simulink model "map_usage"  (R2024b)
settings: Solver=ode1  StartTime=0.0  StopTime=inf  FixedStep=0.01  RelTol=1e-3  EnableMultiTasking=on
PostLoadFcn:
  | qlabs_setup
model workspace (MAT data in the model file):
  Sig = Simulink.Signal
  Sig.Dimensions = -1
  Sig.DimensionsMode = 'auto'
  Sig.Complexity = 'auto'
  Sig.SampleTime = -1
  Sig.SamplingMode = 'auto'
  Sig.DataType = 'auto'
  downCamStepSize = Simulink.Parameter
  downCamStepSize.Value = Simulink.data.Expression
  downCamStepSize.Value.ExpressionString = "qc_get_step_size*ceil(1/30/qc_get_step_size)"
  downCamStepSize.Complexity = 'real'
  downCamStepSize.Dimensions = -1
  downCamStepSize.DataType = 'auto'
  lidarStepSize = Simulink.Parameter
  lidarStepSize.Value = Simulink.data.Expression
  lidarStepSize.Value.ExpressionString = "qc_get_step_size*ceil(1/5/qc_get_step_size)"
  lidarStepSize.Complexity = 'real'
  lidarStepSize.Dimensions = -1
  lidarStepSize.DataType = 'auto'
  mainStepSize = Simulink.Parameter
  mainStepSize.Value = Simulink.data.Expression
  mainStepSize.Value.ExpressionString = "qc_get_step_size"
  mainStepSize.Complexity = 'real'
  mainStepSize.Dimensions = -1
  mainStepSize.DataType = 'auto'
  mode = Simulink.Parameter
  mode.Value = 2
  mode.Complexity = 'real'
  mode.Dimensions = [1 1]
  mode.Description = '0 - education speeds via wheel speed commands
    | 1 - education speeds via body speed commands
    | 2 - research speeds via wheel speed commands
    | 3 - research speeds via body speed commands'
  mode.DataType = 'auto'
  realSenseStepSize = Simulink.Parameter
  realSenseStepSize.Value = Simulink.data.Expression
  realSenseStepSize.Value.ExpressionString = "qc_get_step_size*ceil(1/30/qc_get_step_size)"
  realSenseStepSize.Complexity = 'real'
  realSenseStepSize.Dimensions = -1
  realSenseStepSize.DataType = 'auto'
values from neighbouring files (symbols this model uses):
  map = zeros(mapHeight*pointPerMeter, mapWidth*pointPerMeter)    [map_creator.m]    (also in map_creator_real.m)
  obstacles = [obstacles; coordinateX, coordinateY, rayon;]    [init.m]    (also in init1.m; init_V2.m; init_V3.m; map_creator.m = [)
  pointPerMeter = 50    [map_creator.m]    (also in map_creator_real.m)
  waypoints = [ ... (first row only)    [init.m]    (also in init1.m; init_V2.m; init_V3.m)
undefined symbols (not defined in the file or in its folder): Point
libraries: quarc_library x9, simulink_extras x2
settings Model: ExtModeTrigDuration=10000  Creator=mbohra  LastModifiedBy=simon
settings SolverCC: PositivePriorityOrder=on  AutoInsertRateTranBlk=on
settings DebuggingCC: UnderspecifiedInitializationDetection=Classic  MergeDetectMultiDrivingBlocksExec=none
settings ModelReferenceCC: PropagateSignalLabelsOutOfModel=off
settings RTWCC: Description=QUARC Win64 Target Using Toolchain  SystemTargetFile=quarc_win64.tlc  Toolchain=QUARC win64 | nmake (64-bit Windows)  BuildConfiguration=Faster Runs  GPUComputeCapability=3.5
settings STFCustomTargetCC: TargetLangStandard=C99 (ISO)  ConcurrentExecutionCompliant=on  GRTInterface=on  UseToolchainInfoCompliant=on  SystemTargetFile=quarc_win64.tlc
settings GRTTargetCC: ParMdlRefBuildCompliant=off  CompOptLevelCompliant=off  CombineOutputUpdateFcns=off  MatFileLogging=off  CPPClassGenCompliant=off  GRTInterface=on  ExtMode=on  ExtModeMexFile=quarc_comm

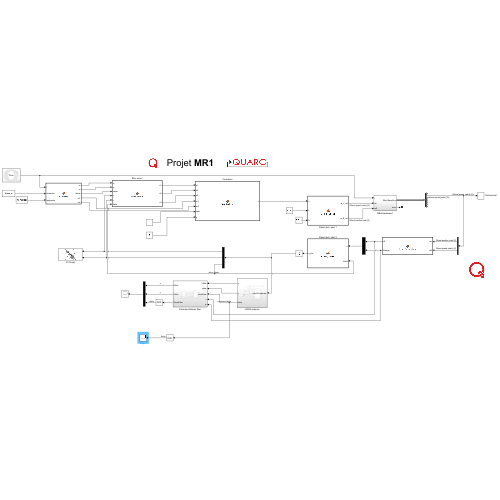
[thumbnail: Simulink's stored preview of the top-level diagram]
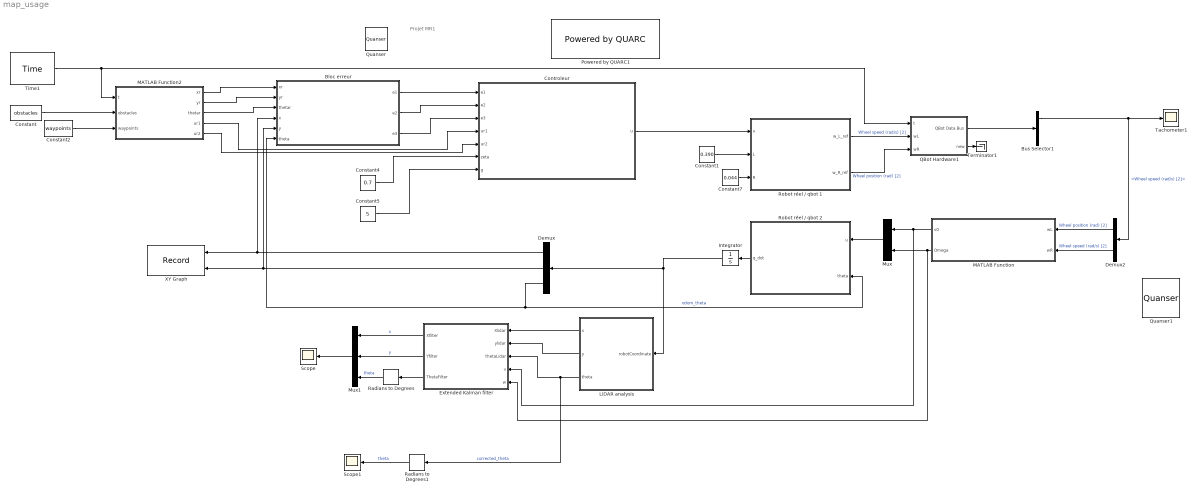
== system map_usage ==
  note: Projet MR1
  Bloc erreur : MATLAB Function  TreatAsAtomicUnit=on
  Bus Selector1 : BusSelector  OutputSignals=Wheel position (rad) [2],Wheel speed (rad/s) [2],Motor Cmd (Volts) [2],Acceleration (m/s/s) [3],Gyroscope (rad/s) [3],Current (Amps) [2],Battery (Volts)
  Constant : Constant  Value=obstacles
  Constant1 : Constant  Value=0.390
  Constant2 : Constant  Value=waypoints
  Constant4 : Constant  Value=0.7
  Constant5 : Constant  Value=5
  Constant7 : Constant  Value=0.044
  Controleur : MATLAB Function  TreatAsAtomicUnit=on
  Demux : Demux  Outputs=3
  Demux2 : Demux  Outputs=2
  Extended Kalman filter : Subsystem
  Integrator : Integrator
  LiDAR analysis : Subsystem
  MATLAB Function : MATLAB Function  TreatAsAtomicUnit=on
  MATLAB Function2 : MATLAB Function  TreatAsAtomicUnit=on
  Mux : Mux  Inputs=2
  Mux1 : Mux  Inputs=3
  Powered by QUARC1 : quarc_library/Logos/Powered by QUARC
  QBot Hardware1 : Subsystem
  Quanser : quarc_library/Logos/Quanser
  Quanser1 : quarc_library/Logos/Quanser
  Radians to Degrees : simulink_extras/Transformations/Radians to Degrees
  Radians to Degrees1 : simulink_extras/Transformations/Radians to Degrees
  Robot réel / qbot 1 : MATLAB Function  TreatAsAtomicUnit=on
  Robot réel / qbot 2 : MATLAB Function  TreatAsAtomicUnit=on
  Scope : Scope
  Scope1 : Scope
  Tachometer1 : Scope
  Terminator1 : Terminator
  Time1 : quarc_library/Sources/Time/Time  time_source=Wall clock  sample_time=qc_get_step_size
  XY Graph : Record  FileSettingsInternal="{\"entries\":[{\"content\":{\"excelSettings\":{\"content\":{},\"type\":\"Streamout.ExcelSettings\"}},\"type\":\"Streamout.FileSettingStorage\",\"uuid\":\"\"}],\"packageUris\":[\"http:\\/\\/schema.mathworks.com\\/mf0\\/streamout_blocks\\/R2020a\"],\"version\":\"1.0\"}"  Layout=[1 1]  SignalsInternal="{\"entries\":[{\"content\":{\"signals\":[{\"content\":{\"blockPath\":[],\"dimensions\":[1,1],\"domain\":\"\",\"lineColor\":\"#a2142f\",\"plots\":[ 1 ],\"port\":1,\"signalID\":1,\"signalName\":\"Demux:1\"},\"type\":\"RecordBlkView.Signal\",\"uuid\":\"\"},{\"content\":{\"blockPath\":[],\"dimensions\":[1,1],\"domain\":\"\",\"lineColor\":\"#139fff\",\"plots\":[ 1 ],\"port\":2,\"signalID\":2,\"signalName\":\"Demux:2\"},\"type\":\"RecordBlkView.Signal\",\"uuid\":\"\"}]},\"type\":\"RecordBlkView.InputSignals\",\"uuid\":\"\"}],\"packageUris\":[\"http:\\/\\/schema.mathworks.com\\/mf0\\/streamout_blocks\\/R2020a\"],\"version\":\"1.0\"}"  VisualizationBindings="{\"xyplotplugin\":{\"info\":[{\"series\":[{\"bindingParametersList\":[{\"parameter\":\"X-Axis\",\"signalID\":1,\"signalName\":\"Demux:1\"},{\"parameter\":\"Y-Axis\",\"signalID\":2,\"signalName\":\"Demux:2\"}],\"seriesID\":0}],\"subplotID\":1}]}}"  CompatibilityTag=XY
  wires:
  Controleur/1(u) -> Robot réel / qbot 1/1(u)
  Constant4/1 -> Controleur/6(zeta)
  Demux/3 -> Robot réel / qbot 2/2(theta), Bloc erreur/6(theta)  "odom_theta"
  Robot réel / qbot 2/1(q_dot) -> Integrator/1
  Bloc erreur/1(e1) -> Controleur/1(e1)
  Demux2/1 -> MATLAB Function/1(wL)  "Wheel position (rad) [2]"
  Demux2/2 -> MATLAB Function/2(wR)  "Wheel speed (rad/s) [2]"
  MATLAB Function/2(Omega) -> Extended Kalman filter/5(w), Mux/2
  Constant1/1 -> Robot réel / qbot 1/2(L)
  Robot réel / qbot 1/1(w_L_ref) -> QBot Hardware1/2(wL)  "Wheel speed (rad/s) [2]"
  Constant5/1 -> Controleur/7(g)
  MATLAB Function2/4(ur1) -> Controleur/4(ur1)
  Time1/1 -> QBot Hardware1/1(t), MATLAB Function2/1(t)
  MATLAB Function/1(v0) -> Extended Kalman filter/4(v), Mux/1
  QBot Hardware1/2(new) -> Terminator1/1
  Bus Selector1/2 -> Demux2/1, Tachometer1/1  "<Wheel speed (rad/s) [2]>"
  MATLAB Function2/1(xr) -> Bloc erreur/1(xr)
  MATLAB Function2/5(ur2) -> Controleur/5(ur2)
  Integrator/1 -> LiDAR analysis/1(robotCoordinate), Demux/1
  Bloc erreur/2(e2) -> Controleur/2(e2)
  Bloc erreur/3(e3) -> Controleur/3(e3)
  Demux/1 -> Bloc erreur/4(x), XY Graph/1
  QBot Hardware1/1(QBot Data Bus) -> Bus Selector1/1
  Robot réel / qbot 1/2(w_R_ref) -> QBot Hardware1/3(wR)  "Wheel position (rad) [2]"
  Constant7/1 -> Robot réel / qbot 1/3(R)
  MATLAB Function2/2(yr) -> Bloc erreur/2(yr)
  MATLAB Function2/3(thetar) -> Bloc erreur/3(thetar)
  Mux/1 -> Robot réel / qbot 2/1(u)
  Constant/1 -> MATLAB Function2/2(obstacles)
  Constant2/1 -> MATLAB Function2/3(waypoints)
  Demux/2 -> Bloc erreur/5(y), XY Graph/2
  LiDAR analysis/1(x) -> Extended Kalman filter/1(Xlidar)
  LiDAR analysis/2(y) -> Extended Kalman filter/2(ylidar)
  LiDAR analysis/3(theta) -> Radians to Degrees1/1, Extended Kalman filter/3(thetaLidar)  "corrected_theta"
  Extended Kalman filter/1(Xfilter) -> Mux1/1  "x"
  Extended Kalman filter/2(Yfilter) -> Mux1/2  "y"
  Extended Kalman filter/3(ThetaFilter) -> Radians to Degrees/1
  Mux1/1 -> Scope/1
  Radians to Degrees/1 -> Mux1/3  "theta"
  Radians to Degrees1/1 -> Scope1/1  "theta"

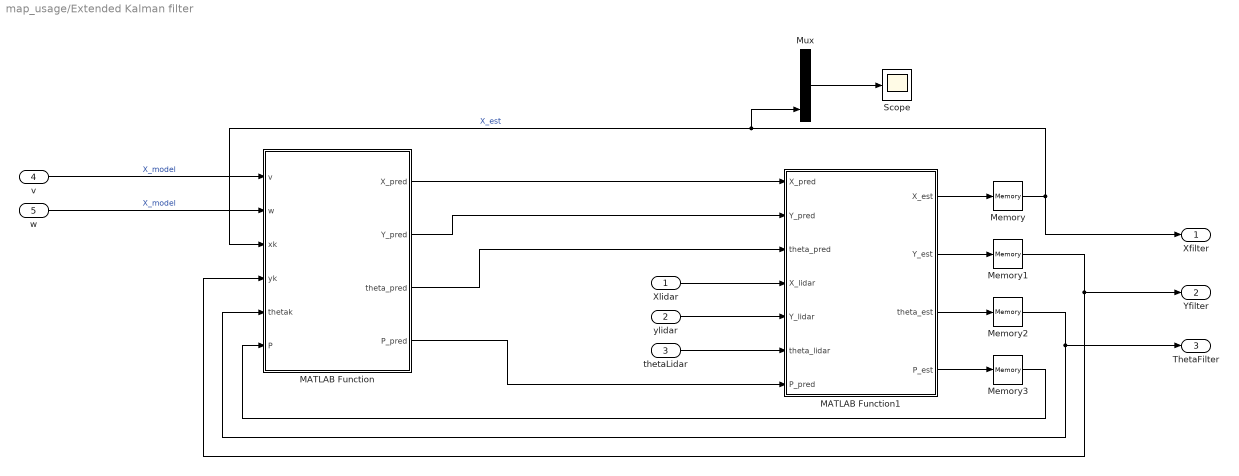
== system map_usage/Extended Kalman filter ==
  Xlidar : Inport
  ylidar : Inport  Port=2
  thetaLidar : Inport  Port=3
  v : Inport  Port=4
  w : Inport  Port=5
  MATLAB Function : MATLAB Function  TreatAsAtomicUnit=on
  MATLAB Function1 : MATLAB Function  TreatAsAtomicUnit=on
  Memory{,1..3} (4 alike) : Memory
  Mux : Mux  Inputs=3
  Scope : Scope
  Xfilter : Outport
  Yfilter : Outport  Port=2
  ThetaFilter : Outport  Port=3
  wires:
  MATLAB Function1/3(theta_est) -> Memory2/1
  MATLAB Function/2(Y_pred) -> MATLAB Function1/2(Y_pred)
  MATLAB Function1/4(P_est) -> Memory3/1
  MATLAB Function/1(X_pred) -> MATLAB Function1/1(X_pred)
  Memory/1 -> Mux/3, MATLAB Function/3(xk), Xfilter/1  "X_est"
  Memory2/1 -> MATLAB Function/5(thetak), ThetaFilter/1
  MATLAB Function1/1(X_est) -> Memory/1
  MATLAB Function/4(P_pred) -> MATLAB Function1/7(P_pred)
  MATLAB Function/3(theta_pred) -> MATLAB Function1/3(theta_pred)
  v/1 -> MATLAB Function/1(v)  "X_model"
  Memory3/1 -> MATLAB Function/6(P)
  Memory1/1 -> MATLAB Function/4(yk), Yfilter/1
  MATLAB Function1/2(Y_est) -> Memory1/1
  Mux/1 -> Scope/1
  Xlidar/1 -> MATLAB Function1/4(X_lidar)
  ylidar/1 -> MATLAB Function1/5(Y_lidar)
  thetaLidar/1 -> MATLAB Function1/6(theta_lidar)
  w/1 -> MATLAB Function/2(w)  "X_model"

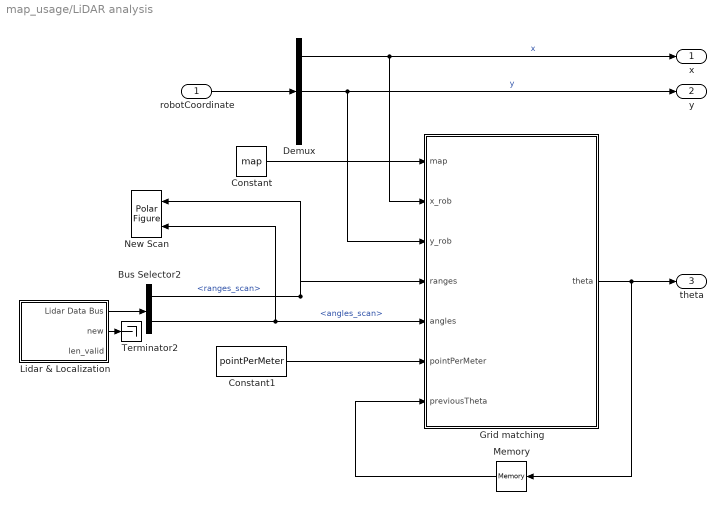
== system map_usage/LiDAR analysis ==
  robotCoordinate : Inport
  Bus Selector2 : BusSelector  OutputSignals=ranges_scan,angles_scan
  Constant : Constant  Value=map
  Constant1 : Constant  Value=pointPerMeter
  Demux : Demux  Outputs=3
  Grid matching : MATLAB Function  TreatAsAtomicUnit=on
  Lidar & Localization : Subsystem
  Memory : Memory
  New Scan : quarc_library/Sinks/Figures/Polar Figure  figure_mode=Use figure window  figure_tag=figure1  axes_tag=axes1  plot_mode=Frame-based  minimum_rho=0  maximum_rho=4  minimum_theta=0  maximum_theta=360  zero_location=top  direction=counterclockwise  buffer_size=1  update_rate=1  sample_time=-1  initial_position="520  231  433  389"  initial_visibility=off  line1_style=None  line1_width=0.5  line1_color=[0 0.4470 0.7410]  marker1=Point (.)  marker1_size=6  marker1_edge_color=[0 0.447059 0.741176]  marker1_face_color=[0 0.447059 0.741176]  line2_style=Solid line (-)  line2_width=0.5  line2_color=[0.85098 0.32549 0.0980392]  marker2=None  marker2_size=6  marker2_edge_color=[0.85098 0.32549 0.0980392]  marker2_face_color=[0.85098 0.32549 0.0980392]  line3_style=Solid line (-)  line3_width=0.5  line3_color=[0.929412 0.694118 0.12549]  marker3=None  marker3_size=6  marker3_edge_color=[0.929412 0.694118 0.12549]  marker3_face_color=[0.929412 0.694118 0.12549]  line4_style=Solid line (-)  line4_width=0.5  line4_color=[0.494118 0.184314 0.556863]  marker4=None  marker4_size=6  marker4_edge_color=[0.494118 0.184314 0.556863]  marker4_face_color=[0.494118 0.184314 0.556863]  line5_style=Solid line (-)  line5_width=0.5  line5_color=[0.466667 0.67451 0.188235]  marker5=None  marker5_size=6  marker5_edge_color=[0.466667 0.67451 0.188235]  marker5_face_color=[0.466667 0.67451 0.188235]
      settings: SourceProductName=QUARC Targets
  Terminator2 : Terminator
  x : Outport
  y : Outport  Port=2
  theta : Outport  Port=3
  wires:
  Constant/1 -> Grid matching/1(map)
  Demux/2 -> Grid matching/3(y_rob), y/1  "y"
  Demux/1 -> Grid matching/2(x_rob), x/1  "x"
  robotCoordinate/1 -> Demux/1
  Grid matching/1(theta) -> theta/1, Memory/1
  Lidar & Localization/1(Lidar Data Bus) -> Bus Selector2/1
  Lidar & Localization/2(new) -> Terminator2/1
  Bus Selector2/2 -> Grid matching/5(angles), New Scan/2  "<angles_scan>"
  Bus Selector2/1 -> Grid matching/4(ranges), New Scan/1  "<ranges_scan>"
  Constant1/1 -> Grid matching/6(pointPerMeter)
  Memory/1 -> Grid matching/7(previousTheta)

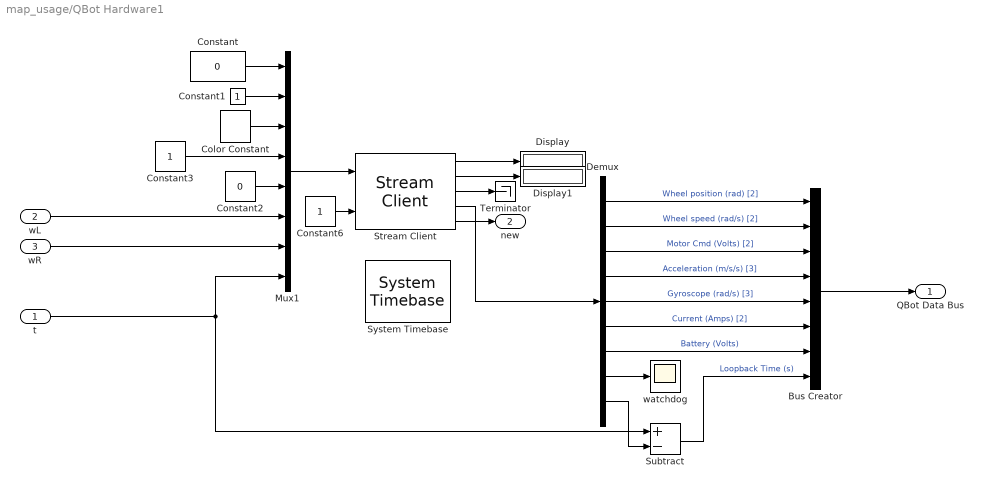
== system map_usage/QBot Hardware1 ==
  t : Inport
  wL : Inport  Port=2
  wR : Inport  Port=3
  Bus Creator : BusCreator  Inputs=8
  Color Constant : quarc_library/Sources/Signals/Color Constant  color=[1 0.07451 0.65098]
      settings: SourceProductName=QUARC Targets
  Constant : Constant  Value=0
  Constant1 : Constant
  Constant2 : Constant  Value=0
  Constant3 : Constant
  Constant6 : Constant
  Demux : Demux  Outputs=[2 2 2 3 3 2 1 1 1]
  Display : Display
  Display1 : Display
  Mux1 : Mux  Inputs=8
  Stream Client : quarc_library/Communications/Basic/Stream Client  uri_source=Specify via dialog (do not evaluate)  uri=tcpip://localhost:18888  send_buffer_size=1460  receive_buffer_size=1460  byte_order=little endian (Intel - LSB first)  optimization=Minimum latency  send_options=Send most recent data  receive_options=Receive most recent data  default_value=zeros(17,1)  sample_time=qc_get_step_size  active=on  implementation=Use blocking I/O in a separate thread  send_fifo_size=1000  receive_fifo_size=1000  send_priority=0  receive_priority=0  send_dimensions=off  receive_dimensions=off  max_dimensions=-1  data_type=Inherited via back propagation  type_expr=BusObject
      settings: AttributesFormatString="\"tcpip://localhost:18888\""
  Subtract : Sum  Inputs=+-
  System Timebase : quarc_library/Advanced/Timing/System Timebase  stop_on_overrun=off
      settings: SourceProductName=QUARC Targets
  Terminator : Terminator
  watchdog : Scope
  QBot Data Bus : Outport
  new : Outport  Port=2
  wires:
  Demux/2 -> Bus Creator/2  "Wheel speed (rad/s) [2]"
  Constant/1 -> Mux1/1
  Stream Client/3 -> Terminator/1
  Stream Client/1 -> Display/1
  Constant6/1 -> Stream Client/2
  Stream Client/2 -> Display1/1
  Color Constant/1 -> Mux1/3
  Constant1/1 -> Mux1/2
  Demux/3 -> Bus Creator/3  "Motor Cmd (Volts) [2]"
  Mux1/1 -> Stream Client/1
  Stream Client/4 -> Demux/1
  Demux/1 -> Bus Creator/1  "Wheel position (rad) [2]"
  Stream Client/5 -> new/1
  Demux/7 -> Bus Creator/7  "Battery (Volts)"
  Demux/5 -> Bus Creator/5  "Gyroscope (rad/s) [3]"
  Demux/6 -> Bus Creator/6  "Current (Amps) [2]"
  Demux/9 -> Subtract/2
  Constant2/1 -> Mux1/5
  Demux/4 -> Bus Creator/4  "Acceleration (m/s/s) [3]"
  t/1 -> Subtract/1, Mux1/8
  Bus Creator/1 -> QBot Data Bus/1
  Subtract/1 -> Bus Creator/8  "Loopback Time (s)"
  Demux/8 -> watchdog/1
  Constant3/1 -> Mux1/4
  wL/1 -> Mux1/6
  wR/1 -> Mux1/7

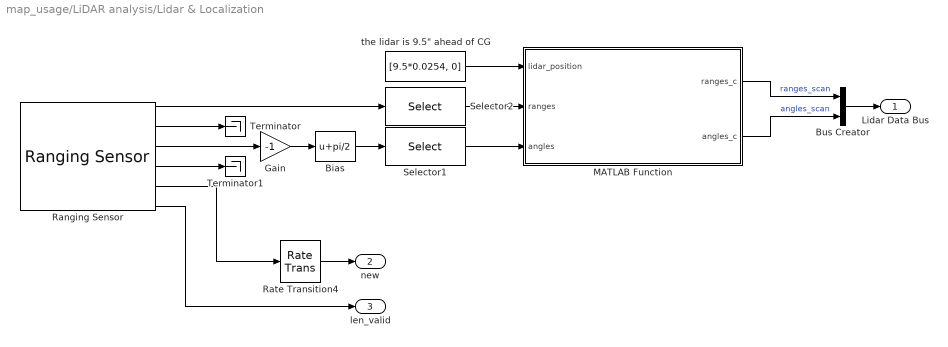
== system map_usage/LiDAR analysis/Lidar & Localization ==
  Bias : Bias  Bias=pi/2  SaturateOnIntegerOverflow=off
  Bus Creator : BusCreator  Inputs=2
  Gain : Gain  Gain=-1
  MATLAB Function : MATLAB Function  TreatAsAtomicUnit=on
  Ranging Sensor : quarc_library/Devices/Third-Party/Sensors/Ranging Sensor  sensor_type=Leishen M10P LIDAR  uri=tcpip://localhost:18918  ranging_distance=Short  timing_budget=0.033  measurement_period=0.0005  output_mode=Fixed-size output  samples_per_revolution=1680  max_distance=0.050  max_angle=5  sample_time=lidarStepSize  show_versions=off  active=on
      settings: SourceProductName=QUARC Targets
  Rate Transition4 : RateTransition
  Selector1 : Selector  InputPortWidth=1680  IndexOptions=Index vector (dialog)  Indices=[1:4:1677]  OutputSizes=1
  Selector2 : Selector  InputPortWidth=1680  IndexOptions=Index vector (dialog)  Indices=[1:4:1677]  OutputSizes=1
  Terminator : Terminator
  Terminator1 : Terminator
  "the lidar is 9.5\" ahead of CG" : Constant  Value=[9.5*0.0254, 0]  SampleTime=lidarStepSize
  Lidar Data Bus : Outport
  new : Outport  Port=2
  len_valid : Outport  Port=3
  wires:
  Ranging Sensor/5 -> Rate Transition4/1
  Rate Transition4/1 -> new/1
  Selector1/1 -> MATLAB Function/3(angles)
  Selector2/1 -> MATLAB Function/2(ranges)
  "the lidar is 9.5\" ahead of CG"/1 -> MATLAB Function/1(lidar_position)
  Bias/1 -> Selector1/1
  Ranging Sensor/2 -> Terminator/1
  Ranging Sensor/4 -> Terminator1/1
  Gain/1 -> Bias/1
  Ranging Sensor/3 -> Gain/1
  Ranging Sensor/1 -> Selector2/1
  MATLAB Function/1(ranges_c) -> Bus Creator/1  "ranges_scan"
  MATLAB Function/2(angles_c) -> Bus Creator/2  "angles_scan"
  Bus Creator/1 -> Lidar Data Bus/1
  Ranging Sensor/6 -> len_valid/1

== matlab function map_usage/Controleur ==
  data: e1 input; e2 input; e3 input; u output; ur1 input; ur2 input; zeta input; g input
function u = Controlleur(e1, e2, e3, ur1, ur2, zeta, g)

    % Gain Scheduling + équation 1_ et 19

        wn = sqrt(ur2^2 + g*ur1^2);

        % Calcul des gains
        k1 = 2*zeta*wn;
        k3 = k1;                        % dans l'équation 15, k1 = k3
        k2 = g*abs(ur1);                % gain variable selon la vitesse
    
    % Calcul des corrections feedback -> équatioon 11
        v1 = -k1 * e1;
        v2 = -sign(ur1)*k2*e2 - k3*e3;
        % v1 = 0;
        % v2 = 0;

    % Commande totaleuuuu Feedforward + Feedback -> équation 7
        u1 = ur1 *cos(e3) - v1;
        u2 = ur2 - v2;
        

        u = [u1; u2];
end

== matlab function map_usage/MATLAB Function ==
  data: wL input; v0 output; wR input; Omega output
function [v0, Omega] = Fwd_Kinematics(wL, wR)
    % wL : Vitesse angulaire roue gauche (rad/s)
    % wR : Vitesse angulaire roue droite (rad/s)
    % R  : Rayon de la roue (m)
    % L  : Entraxe (distance entre les roues en m)

    R = 0.044;   % Rayon de la roue (44 mm)
    L = 0.390;   % Entraxe entre les roues (39 cm)

    % 1. Conversion en vitesse linéaire de chaque roue (m/s)
    v_left = wL * R;
    v_right = wR * R;

    % 2. Calcul de la vitesse linéaire du robot (v0)
    % C'est la moyenne des deux roues
    v0 = (v_right + v_left) / 2;

    % 3. Calcul de la vitesse de rotation du robot (Omega)
    % C'est la différence de vitesse divisée par la largeur du robot
    Omega = (v_right - v_left) / L;
    
end

== matlab function map_usage/Robot réel // qbot 1 ==
  data: w_L_ref output; u input; w_R_ref output; L input; R input
function [w_L_ref, w_R_ref] = Motors_Speed(u, L, R)
    % u(1) = u1 (Vitesse linéaire v en m/s)
    % u(2) = u2 (Vitesse angulaire omega en rad/s)

    v = u(1);
    omega = u(2);

    % Calcul des vitesses linéaires de chaque roue 
    w_L_ref = (2*v-L*omega)/(2*R);
    w_R_ref = (2*v+L*omega)/(2*R);
    % Conversion en vitesse angulaire (rad/s) pour les moteurs
    %w_R_ref = (v_R / R);
    %w_L_ref = (v_L / R);
end

== matlab function map_usage/Robot réel // qbot 2 ==
  data: u input; q_dot output; theta input
function q_dot  = Robot_Model(u, theta)
    % u(1) = u1 (vitesse linéaire)
    % u(2) = u2 (vitesse angulaire)

    q_dot = [0;0;0];
    q_dot(1) = u(1) * cos(theta);
    q_dot(2) = u(1) * sin(theta);
    q_dot(3) = u(2);
end

== matlab function map_usage/LiDAR analysis/Grid matching ==
  data: map input; x_rob input; y_rob input; ranges input; angles input; theta output double; pointPerMeter input; previousTheta input
function theta = estimate_theta(map, x_rob, y_rob, ranges, angles, pointPerMeter, previousTheta)
    %#codegen
    % Note : x_rob et y_rob représentent ici la position du LiDAR, 
    % l'offset ayant été géré en amont dans le schéma Simulink.
    
    % --- Paramètres ---
    [mapRows, mapCols] = size(map);
    % On suppose que le centre de la matrice correspond aux coordonnées (0,0)
    center_row = mapRows / 2;
    center_col = mapCols / 2;
    
    % --- Filtrage des mesures LiDAR ---
    valid_idx = (ranges > 0) & (ranges < inf);
    r_valid = ranges(valid_idx);
    a_valid = angles(valid_idx);
    
    % --- Recherche de l'angle optimal (Scan Matching) ---
    % Test des angles de -pi à pi avec une résolution de 1 degré
    theta_search = -pi : (pi/180) : pi; 
    
    best_score = -1;
    best_theta = 0;
    
    % Boucle sur chaque angle possible
    for i = 1:length(theta_search)
        t = theta_search(i);
        
        % 1. Projection des points LiDAR dans le repère global
        % L'angle global du rayon est l'angle local du LiDAR + l'angle testé (t)
        x_pts = x_rob + r_valid .* cos(a_valid + t);
        y_pts = y_rob + r_valid .* sin(a_valid + t);
        
        % 2. Conversion des coordonnées monde (m) en indices de matrice (pixels)
        cols = round(center_col + (x_pts * pointPerMeter));
        rows = round(center_row - (y_pts * pointPerMeter)); 
        
        % 3. Filtrage de sécurité : on ignore les points hors de la carte
        in_bounds = (rows >= 1) & (rows <= mapRows) & (cols >= 1) & (cols <= mapCols);
        rows_in = rows(in_bounds);
        cols_in = cols(in_bounds);
        
        % 4. Calcul du score
        if isempty(rows_in)
            score = 0;
        else
            % Score = somme des "probabilités" d'obstacle sur la carte
            linear_indices = sub2ind([mapRows, mapCols], rows_in, cols_in);
            score = sum(map(linear_indices));
        end
        
        % 5. Mémorisation du meilleur angle
        if score > best_score
            best_score = score;
            best_theta = t;
        end
    end
    
    % Sortie finale (seulement si le theta est cohérent)
    difference = rad2deg(previousTheta-best_theta);
    if difference >= -45 && difference <= 45
        theta = best_theta;
    else
        theta = previousTheta;
    end
end

== matlab function map_usage/MATLAB Function2 ==
  data: t input; xr output; yr output; thetar output; ur1 output; ur2 output; obstacles input; waypoints input
function [xr, yr, thetar, ur1, ur2] = Traj_bezier3(t, obstacles, waypoints)
    % Entrée : t (temps de simulation)
    % Sorties : Références x, y, theta, v, omega

    coder.extrinsic('plot');

    % Mémoire pour stocker la trajectoire calculée une seule fois
    persistent time_ref x_ref y_ref theta_ref v_ref omega_ref initialized
    
    if isempty(initialized)
        v_max = 0.5;           
        omega_max = 2.0;       
                
        % Obstacles Rectangulaires [x, y, w, h, theta]
        obstacles_rect = [
            %1.0, 1.0, 2.0, 1, 0;    
        ];

        gates = [];
        n_points_per_seg = 1000; % Points par segment
        marge_securite = 0.5;

        % Initialisation des vecteurs totaux
        x_total = []; y_total = []; theta_total = [];
        v_total = []; omega_total = []; time_total = [];
        
        cumul_time = 0;
        
        % Boucle sur chaque segment (entre waypoint i et i+1)
        for seg = 1:(size(waypoints, 1) - 1)
            
            x_start = waypoints(seg, 1); y_start = waypoints(seg, 2); theta_start = waypoints(seg, 3);
            x_goal = waypoints(seg+1, 1); y_goal = waypoints(seg+1, 2); theta_goal = waypoints(seg+1, 3);
            
            % Tangentes -> points intermédiaires
            distance = sqrt((x_goal - x_start)^2 + (y_goal - y_start)^2);
            longueur_tangente = distance / 3;
             
            P0 = [x_start, y_start];
            P1 = P0 + longueur_tangente * [cos(theta_start), sin(theta_start)];
            P2 = [x_goal, y_goal] - longueur_tangente * [cos(theta_goal), sin(theta_goal)];
            P3 = [x_goal, y_goal];
            
            % On modifie les points intermédiaires s'ils sont trop proche
            % d'un obstacle
            for i = 1:size(obstacles, 1)
                obs_c = obstacles(i, 1:2); r_obs = obstacles(i, 3);
                
                % P1
                if norm(P1 - obs_c) < r_obs + marge_securite + 0.5
                    dir = (P1 - obs_c) / norm(P1 - obs_c);
                    P1 = obs_c + dir * (r_obs + marge_securite + 0.8);
                end
                % P2
                if norm(P2 - obs_c) < r_obs + marge_securite + 0.5
                    dir = (P2 - obs_c) / norm(P2 - obs_c);
                    P2 = obs_c + dir * (r_obs + marge_securite + 0.8);
                end
            end
            
            for i = 1:size(obstacles_rect, 1)
                xc = obstacles_rect(i, 1); yc = obstacles_rect(i, 2);
                W = obstacles_rect(i, 3); H = obstacles_rect(i, 4); ang = obstacles_rect(i, 5);
                R_mat = [cos(ang), -sin(ang); sin(ang), cos(ang)];
                corners_loc = [-W/2, -H/2; W/2, -H/2; W/2, H/2; -W/2, H/2];
                corners_glob = (R_mat * corners_loc')' + [xc, yc];
                r_coin = 0.3;
                
                % Vérifier P1 et P2 contre les 4 coins
                for j=1:4
                    coin = corners_glob(j,:);
                    if norm(P1 - coin) < r_coin + marge_securite + 0.5
                         dir = (P1 - coin)/norm(P1 - coin);
                         P1 = coin + dir * (r_coin + marge_securite + 0.8);
                    end
                    if norm(P2 - coin) < r_coin + marge_securite + 0.5
                         dir = (P2 - coin)/norm(P2 - coin);
                         P2 = coin + dir * (r_coin + marge_securite + 0.8);
                    end
                end
            end
            
            % génération de la trajectoire via Bezier
            tt = linspace(0, 1, n_points_per_seg)';
            x_seg = (1-tt).^3*P0(1) + 3*(1-tt).^2.*tt*P1(1) + 3*(1-tt).*tt.^2*P2(1) + tt.^3*P3(1);
            y_seg = (1-tt).^3*P0(2) + 3*(1-tt).^2.*tt*P1(2) + 3*(1-tt).*tt.^2*P2(2) + tt.^3*P3(2);
            

            dx = gradient(x_seg); dy = gradient(y_seg);
            theta_seg = atan2(dy, dx);
            
            ddx = gradient(dx); ddy = gradient(dy);
            kappa = (dx.*ddy - dy.*ddx) ./ (dx.^2 + dy.^2).^(3/2);
            kappa(isnan(kappa)) = 0;
            
            % Profil de vitesse
            v_seg = v_max * ones(size(kappa));
            for k=1:length(kappa)
                if abs(kappa(k)) > 0.01 % si la courbure est trop elevee on ralentit
                    v_lim = sqrt(3.0 / abs(kappa(k)));
                    v_seg(k) = min(v_seg(k), v_lim);
                end
            end
            v_seg = min(v_seg, v_max);
            
            omega_seg = v_seg .* kappa;
            omega_seg = max(min(omega_seg, omega_max), -omega_max);
            
            % conversion du temps de bezier ([0,1]) en un temps reel base
            % sur le calcul du temp total
            ds = sqrt(diff(x_seg).^2 + diff(y_seg).^2);
            ds = [0; ds];
            dt = ds ./ max(v_seg, 0.01);
            time_seg = cumsum(dt) + cumul_time;

            if seg == 1
                x_total = [x_total; x_seg];
                y_total = [y_total; y_seg];
                theta_total = [theta_total; theta_seg];
                v_total = [v_total; v_seg];
                omega_total = [omega_total; omega_seg];
                time_total = [time_total; time_seg];
            else
                % On saute le premier point pour éviter les doublons
                x_total = [x_total; x_seg(2:end)];
                y_total = [y_total; y_seg(2:end)];
                theta_total = [theta_total; theta_seg(2:end)];
                v_total = [v_total; v_seg(2:end)];
                omega_total = [omega_total; omega_seg(2:end)];
                time_total = [time_total; time_seg(2:end)];
            end
            
            cumul_time = time_total(end);
        end
        
        % Correction finale des angles (Unwrap) pour éviter les sauts +/- Pi
        theta_total = unwrap(theta_total);

        % Stockage Persistant
        time_ref = time_total;
        x_ref = x_total;
        y_ref = y_total;
        theta_ref = theta_total;
        v_ref = v_total;
        omega_ref = omega_total;

        figure('Name', 'Trajectoire Bézier Multi-Points', 'Position', [970 100 900 700]);
        hold on; grid on; axis equal;
        
        % Dessiner obstacles circulaires
        for i = 1:size(obstacles, 1)
            circle_x = obstacles(i,1) + obstacles(i,3) * cos(0:0.01:2*pi);
            circle_y = obstacles(i,2) + obstacles(i,3) * sin(0:0.01:2*pi);
            fill(circle_x, circle_y, [1 0.7 0.7], 'EdgeColor', 'r', 'LineWidth', 2);
        end

        % Dessiner la trajectoire complète
        plot(x_ref, y_ref, 'b-', 'LineWidth', 3);
        
        % Dessiner les waypoints
        for i = 1:size(waypoints, 1)
            if i == 1
                % Point de départ (vert)
                plot(waypoints(i,1), waypoints(i,2), 'go', 'MarkerSize', 15, 'MarkerFaceColor', 'g');
                quiver(waypoints(i,1), waypoints(i,2), 0.4*cos(waypoints(i,3)), ...
                       0.4*sin(waypoints(i,3)), 0, 'g', 'LineWidth', 3, 'MaxHeadSize', 1);
            elseif i == size(waypoints, 1)
                % Point d'arrivée final (rouge)
                plot(waypoints(i,1), waypoints(i,2), 'ro', 'MarkerSize', 15, 'MarkerFaceColor', 'r');
                quiver(waypoints(i,1), waypoints(i,2), 0.4*cos(waypoints(i,3)), ...
                       0.4*sin(waypoints(i,3)), 0, 'r', 'LineWidth', 3, 'MaxHeadSize', 1);
            else
                % Points intermédiaires (bleu)
                plot(waypoints(i,1), waypoints(i,2), 'bo', 'MarkerSize', 12, 'MarkerFaceColor', 'b');
                quiver(waypoints(i,1), waypoints(i,2), 0.4*cos(waypoints(i,3)), ...
                       0.4*sin(waypoints(i,3)), 0, 'b', 'LineWidth', 2, 'MaxHeadSize', 1);
            end
        end
        
        initialized = 1;
    end
    
    
    if t > time_ref(end)
        % Fin de la trajectoire : on reste sur place
        xr = x_ref(end);
        yr = y_ref(end);
        thetar = theta_ref(end);
        ur1 = 0; % Vitesse linéaire nulle
        ur2 = 0; % Vitesse angulaire nulle
    else
        % on trouve les valeurs exactes au temp t en interpolant dans les
        % tableaux calcule
        % Interpolation
        xr = interp1(time_ref, x_ref, t, 'spline');
        yr = interp1(time_ref, y_ref, t, 'spline');
        thetar = interp1(time_ref, theta_ref, t, 'spline');
        ur1 = interp1(time_ref, v_ref, t, 'spline');
        ur2 = interp1(time_ref, omega_ref, t, 'spline');
    end
    xfull = x_ref;
    yfull = y_ref;
end

== matlab function map_usage/LiDAR analysis/Lidar & Localization/MATLAB Function ==
  data: lidar_position input; ranges input; ranges_c output; angles input; angles_c output
function [ranges_c,angles_c] = correct_lidar(lidar_position, ranges,angles)

x = ranges.*cos(angles) + lidar_position(1);
y = ranges.*sin(angles) + lidar_position(2);

ranges_c = sqrt(x.^2 + y.^2);
angles_c = atan2(y, x);

end

== matlab function map_usage/Bloc erreur ==
  data: e1 output; xr input; yr input; thetar input; x input; y input; theta input; e2 output; e3 output
function [e1, e2, e3] = Bloc_erreur(xr, yr, thetar, x, y, theta)

    % Calcul des erreurs dans le repère global
    ex_global = xr - x;
    ey_global = yr - y;
    etheta_global = thetar - theta;


    % Normalisation de l'angle de -pi à pi
    etheta_global = atan2(sin(etheta_global), cos(etheta_global));

    % Matrice de Rotattion de l'équation 5 du paper
    e1 =  cos(theta) * ex_global + sin(theta) * ey_global;
    e2 = -sin(theta) * ex_global + cos(theta) * ey_global;
    e3 = etheta_global;

    
end

== matlab function map_usage/Extended Kalman filter/MATLAB Function ==
  data: v input; X_pred output; w input; xk input; yk input; thetak input; P input; Y_pred output; theta_pred output; P_pred output
function [X_pred, Y_pred, theta_pred, P_pred] = prediction(v, w, xk, yk, thetak, P)
    % Vecteur d'état actuel
    X = [xk; yk; thetak];
   
    % 1. MODÈLE D'ÉTAT (Cinématique du QBot)
    % On calcule la prédiction basée sur les vitesses v (linéaire) et w (angulaire)
    X_next = X + [v * cos(thetak);
                  v * sin(thetak);
                  w];
    
    % Extraction des sorties
    X_pred     = X_next(1);
    Y_pred     = X_next(2);
    theta_pred = atan2(sin(X_next(3)), cos(X_next(3))); % Normalisation d'angle (-pi à pi)

    % 2. LINÉARISATION (Calcul de la Jacobienne F)
    % f est la dérivée de l'équation d'état par rapport à x, y et theta
    F = [1, 0, -v * sin(thetak);
         0, 1,  v * cos(thetak);
         0, 0,  1];

    % 3. BRUIT DE MODÈLE (Matrice Q)
    % Plus ces valeurs sont élevées, moins on fait confiance au modèle théorique
    % À ajuster
    q_x = 0.00001; %0.001
    q_y = 0.00001;%0.001
    q_theta = 0.00002;%0.002
    Q = diag([q_x, q_y, q_theta]);

    % 4. PRÉDICTION DE LA COVARIANCE
    % On propage l'incertitude P_pred = F*P*F' + Q
    P_pred = F * P * F' + Q;
end

== matlab function map_usage/Extended Kalman filter/MATLAB Function1 ==
  data: X_pred input; X_est output; Y_pred input; theta_pred input; X_lidar input; Y_lidar input; theta_lidar input; P_pred input; Y_est output; theta_est output; P_est output
function [X_est, Y_est, theta_est, P_est] = update(X_pred, Y_pred, theta_pred, X_lidar, Y_lidar, theta_lidar, P_pred)
    % 1. VECTEURS D'ÉTAT ET DE MESURE
    x_p = [X_pred; Y_pred; theta_pred];
    z = [X_lidar; Y_lidar; theta_lidar];

    % 2. MODÈLE D'OBSERVATION (H)
    % Puisque le LIDAR mesure directement x, y et theta, H est l'identité
    H = eye(3);

    % 3. MATRICE DE BRUIT DE MESURE (R)
    % Plus ces valeurs sont faibles, plus le filtre fera confiance au LIDAR
    % (À ajuster selon la précision du LIDAR)
    r_dist = 0.00005; % Incertitude en mètres 0.05
    r_ang  = 0.00002; % Incertitude en radians0.02
    R = diag([r_dist, r_dist, r_ang]);

    % 4. CALCUL DU GAIN DE KALMAN (K)
    % S est la covariance de l'innovation
    S = H * P_pred * H' + R;
    K = P_pred * H' / S;

    % 5. CALCUL DE L'Erreur entre LIDAR et Prédiction
    innovation = z - (H * x_p);

    %Normalisation de l'erreur d'angle
    % Empêche le filtre de paniquer si le LIDAR dit 179° et le modèle 181° (-179°)
    innovation(3) = atan2(sin(innovation(3)), cos(innovation(3)));

    % 6. MISE À JOUR DE L'ÉTAT ET DE LA COVARIANCE
    x_corrected = x_p + K * innovation;
    P_corrected = (eye(3) - K * H) * P_pred;

    % 7. ASSIGNATION DES SORTIES
    X_est = x_corrected(1);
    Y_est = x_corrected(2);
    theta_est = atan2(sin(x_corrected(3)), cos(x_corrected(3)));
    P_est = P_corrected;
end
